simulink library "Steer_Control_Axle2"  (R2022b)
settings: Solver=VariableStepAuto  StartTime=0.0  StopTime=10.0  RelTol=1e-3
undefined symbols (not defined in the file): Control
libraries: simulink_extras x2
Description:
  | Simscape Vehicle Templates Library
  | 
  | Copyright 2018-2024 The MathWorks, Inc.
settings Model: Creator=smiller  LastModifiedBy=smiller
settings ModelReferenceCC: EnableRefExpFcnMdlSchedulingChecks=on

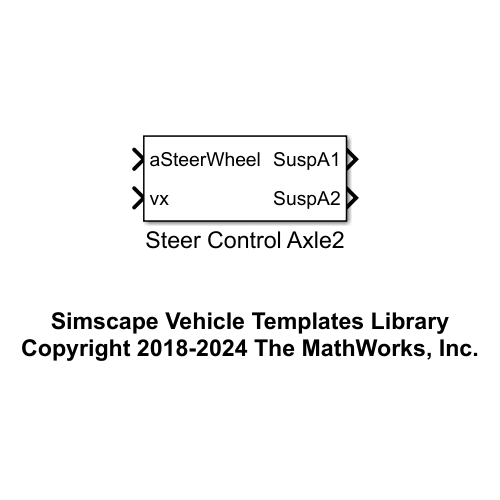
[thumbnail: Simulink's stored preview of the top-level diagram]
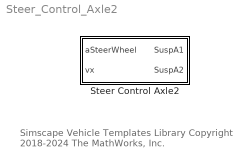
== system Steer_Control_Axle2 ==
  note: Simscape Vehicle Templates Library
      | Copyright 2018-2024 The MathWorks, Inc.
  Steer Control Axle2 : Subsystem  mask(Steer Control, Two Axle){Steer=Control.Default.Steer}
      mask prompts: Steer "Steer (structure)"
      mask help: Steering control for two-axle vehicles.

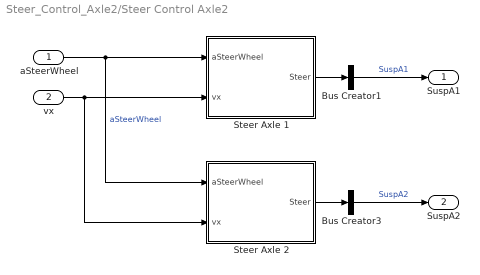
== system Steer_Control_Axle2/Steer Control Axle2 ==
  aSteerWheel : Inport
  vx : Inport  Port=2
  Bus Creator1 : BusCreator  Inputs=1
  Bus Creator3 : BusCreator  Inputs=1
  Steer Axle 1 : Subsystem
  Steer Axle 2 : Subsystem
  SuspA1 : Outport  VectorParamsAs1DForOutWhenUnconnected=off
  SuspA2 : Outport  Port=2  VectorParamsAs1DForOutWhenUnconnected=off
  wires:
  vx/1 -> Steer Axle 1/2(vx), Steer Axle 2/2(vx)
  Bus Creator3/1 -> SuspA2/1  "SuspA2"
  aSteerWheel/1 -> Steer Axle 2/1(aSteerWheel), Steer Axle 1/1(aSteerWheel)  "aSteerWheel"
  Steer Axle 1/1(Steer) -> Bus Creator1/1
  Bus Creator1/1 -> SuspA1/1  "SuspA1"
  Steer Axle 2/1(Steer) -> Bus Creator3/1

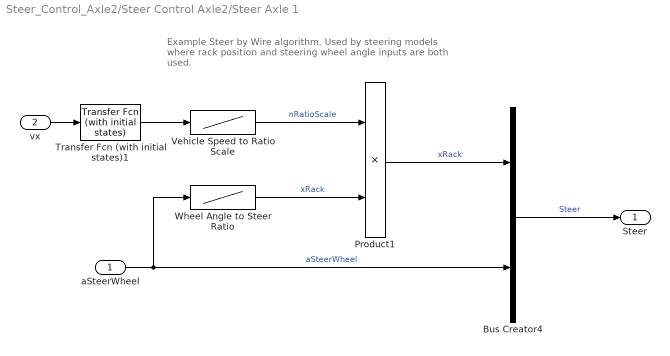
== system Steer_Control_Axle2/Steer Control Axle2/Steer Axle 1 ==
  note: Example Steer by Wire algorithm.
      | Used by steering models where rack position
      | and steering wheel angle inputs are both used.
  aSteerWheel : Inport
  vx : Inport  Port=2
  Bus Creator4 : BusCreator  Inputs=2
  Product1 : Product
  Transfer Fcn (with initial states)1 : simulink_extras/Additional Linear/Transfer Fcn (with initial states)  N=[1]  D="[1/Steer.fActuatorCutoff.Value  1]"  X0=-1
  Vehicle Speed to Ratio Scale : Lookup_n-D  NumberOfTableDimensions=1  BreakpointsForDimension1=Control.Default.Steer.Ratio_Scale.vVehicle.Value  Table=Control.Default.Steer.Ratio_Scale.n.Value  InternalRulePriority=Speed  RndMeth=Simplest
  Wheel Angle to Steer Ratio : Lookup_n-D  NumberOfTableDimensions=1  BreakpointsForDimension1=Control.Default.Steer.Ratio_Table.aWheel.Value  Table=Control.Default.Steer.Ratio_Table.xRack.Value  InternalRulePriority=Speed  RndMeth=Simplest
  Steer : Outport  VectorParamsAs1DForOutWhenUnconnected=off
  wires:
  Bus Creator4/1 -> Steer/1  "Steer"
  vx/1 -> Transfer Fcn (with initial states)1/1
  Product1/1 -> Bus Creator4/1  "xRack"
  Wheel Angle to Steer Ratio/1 -> Product1/2  "xRack"
  aSteerWheel/1 -> Bus Creator4/2, Wheel Angle to Steer Ratio/1  "aSteerWheel"
  Transfer Fcn (with initial states)1/1 -> Vehicle Speed to Ratio Scale/1
  Vehicle Speed to Ratio Scale/1 -> Product1/1  "nRatioScale"

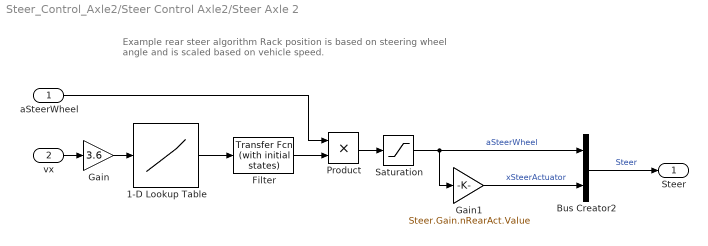
== system Steer_Control_Axle2/Steer Control Axle2/Steer Axle 2 ==
  note: Example rear steer algorithm
      | Rack position is based on steering wheel angle
      | and is scaled based on vehicle speed.
  aSteerWheel : Inport
  vx : Inport  Port=2
  1-D Lookup Table : Lookup_n-D  NumberOfTableDimensions=1  BreakpointsForDimension1=Steer.Gain.vVehicle.Value  Table=Steer.Gain.n.Value  InterpMethod=Linear Lagrange  InternalRulePriority=Speed  RndMeth=Simplest
  Bus Creator2 : BusCreator  Inputs=2
  Filter : simulink_extras/Additional Linear/Transfer Fcn (with initial states)  N=[1]  D="[1/Steer.fActuatorCutoff.Value  1]"  X0=-1
  Gain : Gain  Gain=3.6
  Gain1 : Gain  Gain=Steer.Gain.nRearAct.Value
  Product : Product
  Saturation : Saturate  UpperLimit=Steer.Limits.aUpper.Value  LowerLimit=Steer.Limits.aLower.Value  LinearizeAsGain=off  ZeroCross=off
  Steer : Outport
  wires:
  vx/1 -> Gain/1
  1-D Lookup Table/1 -> Filter/1
  Gain1/1 -> Bus Creator2/2  "xSteerActuator"
  Filter/1 -> Product/2
  Product/1 -> Saturation/1
  Saturation/1 -> Gain1/1, Bus Creator2/1  "aSteerWheel"
  Bus Creator2/1 -> Steer/1  "Steer"
  Gain/1 -> 1-D Lookup Table/1
  aSteerWheel/1 -> Product/1
